simulink model "NOx_Aftertratment"  (R2019a)
settings: Solver=FixedStepDiscrete  StartTime=0.0  StopTime=10.0  RelTol=1e-3
settings Model: Creator=Kore  LastModifiedBy=Kore

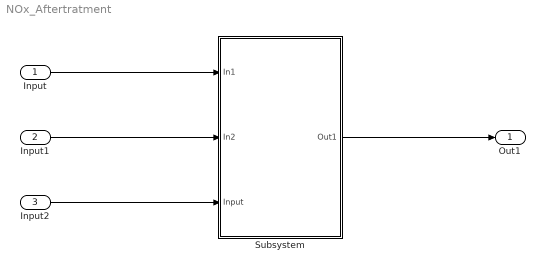
== system NOx_Aftertratment ==
  Input : Inport
  Input1 : Inport  Port=2
  Input2 : Inport  Port=3
  Subsystem : Subsystem
  Out1 : Outport
  wires:
  Input/1 -> Subsystem/1(In1)
  Input1/1 -> Subsystem/2(In2)
  Input2/1 -> Subsystem/3(Input)
  Subsystem/1(Out1) -> Out1/1

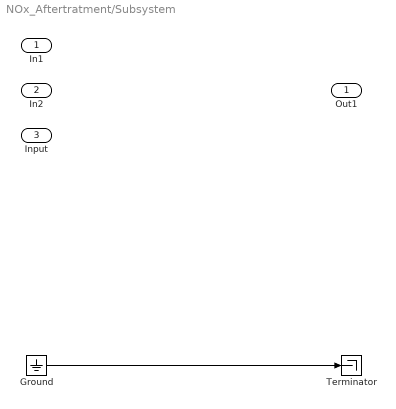
== system NOx_Aftertratment/Subsystem ==
  In1 : Inport
  In2 : Inport  Port=2
  Input : Inport  Port=3
  Ground : Ground
  Terminator : Terminator
  Out1 : Outport
  wires:
  Ground/1 -> Terminator/1
